simulink library "MMC"  (R2018b)
settings: Solver=VariableStepAuto  StartTime=0.0  StopTime=10.0  RelTol=1e-3
libraries: powerlib x4, spsControlledCurrentSourceLib x1, spsCurrentMeasurementLib x1
settings Model: Creator=fcolas  LastModifiedBy=Frederic_Colas
settings DataIOCC: ReturnWorkspaceOutputs=on

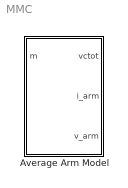
== system MMC ==
  Average Arm Model : Subsystem  mask{C_arm=0, Vdc=0}
      mask prompts: C_arm "Arm equivalent Capacitor (F)"; Vdc "Init DC Voltage (V)"

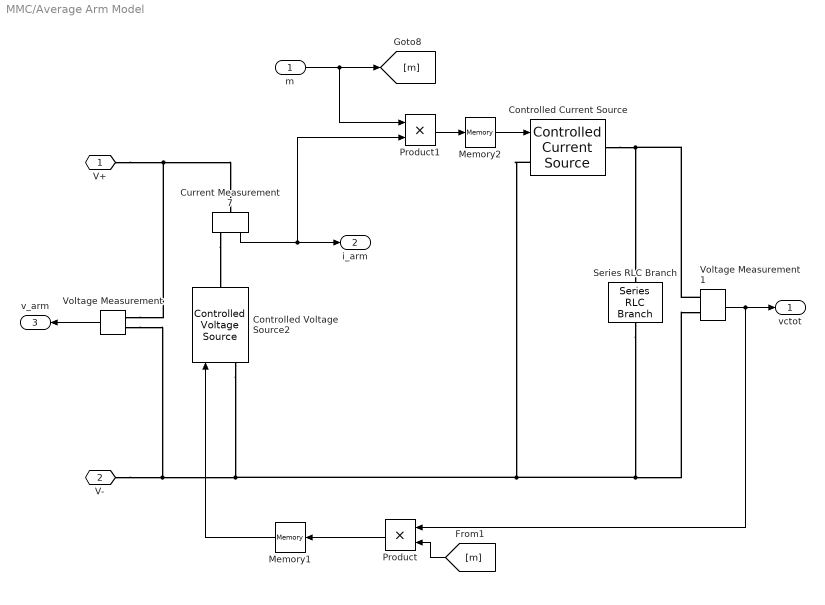
== system MMC/Average Arm Model ==
  m : Inport
  Controlled Current Source : spsControlledCurrentSourceLib/Controlled Current Source  Initialize=on  Source_Type=DC  Amplitude=0  Phase=0  Frequency=0  Measurements=None
  Controlled Voltage Source2 : powerlib/Electrical Sources/Controlled Voltage Source  Initialize=on  Source_Type=DC  Amplitude=Vdc/2  Phase=180  Frequency=0  Measurements=None
  Current Measurement7 : spsCurrentMeasurementLib/Current Measurement  PhasorSimulation=off  OutputType=Complex  PSBequivalent=0
  Memory1 : Memory  InitialCondition=Vdc/2
  Memory2 : Memory
  Product : Product  RndMeth=Zero
  Product1 : Product  RndMeth=Zero
  Series RLC Branch : powerlib/Elements/Series RLC Branch  LConnTagsString=__new0  RConnTagsString=__new0  BranchType=C  Resistance=1  Inductance=1e-3  SetiL0=off  InitialCurrent=0  Capacitance=C_arm  Setx0=on  InitialVoltage=Vdc  Measurements=None
  Voltage Measurement : powerlib/Measurements/Voltage Measurement  PhasorSimulation=off  OutputType=Complex  PSBequivalent=0
  Voltage Measurement1 : powerlib/Measurements/Voltage Measurement  PhasorSimulation=off  OutputType=Complex  PSBequivalent=0
  V+ : PMIOPort  Side=Left
  V- : PMIOPort  Port=2  Side=Left
  vctot : Outport
  i_arm : Outport  Port=2
  v_arm : Outport  Port=3
  wires:
  Voltage Measurement1/1 -> vctot/1, Product/1
  [m] -> Product/2
  Current Measurement7/1 -> Product1/2, i_arm/1
  m/1 -> Product1/1, [m]
  Product1/1 -> Memory2/1
  Voltage Measurement/1 -> v_arm/1
  Product/1 -> Memory1/1
  Memory2/1 -> Controlled Current Source/1
  Memory1/1 -> Controlled Voltage Source2/1
  connections:
  Voltage Measurement1/LConn1 -- Series RLC Branch/LConn1 -- Controlled Current Source/RConn1
  Controlled Voltage Source2/LConn1 -- Voltage Measurement/LConn2 -- V-/RConn1 -- Voltage Measurement1/LConn2 -- Series RLC Branch/RConn1 -- Controlled Current Source/LConn1
  V+/RConn1 -- Voltage Measurement/LConn1 -- Current Measurement7/LConn1
  Current Measurement7/RConn1 -- Controlled Voltage Source2/RConn1
